simulink model "inverter"  (R2021a)
settings: Solver=VariableStepAuto  StartTime=0.0  StopTime=1  RelTol=1e-3
libraries: spsSeriesRLCBranchLib x2, spsDCVoltageSourceLib x1, spsGroundLib x1, spsThreePhaseParallelRLCBranchLib x1, spsPWMGenerator3LevelLib x1, spsThreeLevelBridgeLib x1, spsThreePhaseVIMeasurementLib x1, spspowerguiLib x1
settings Model: Creator=mluser  LastModifiedBy=mluser

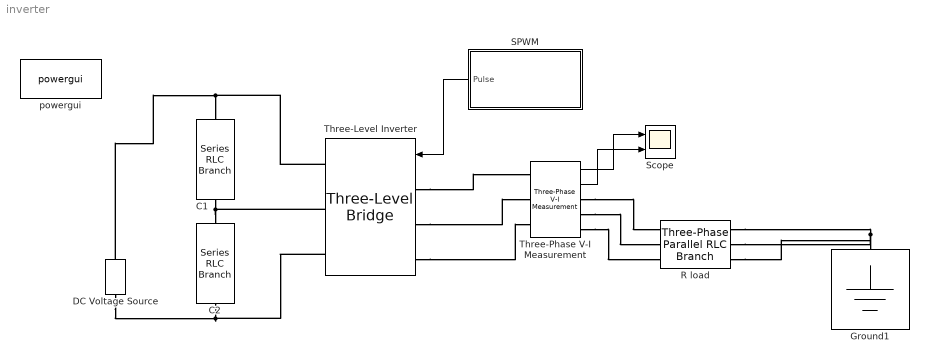
== system inverter ==
  C1 : spsSeriesRLCBranchLib/Series RLC Branch  LConnTagsString=__new0  RConnTagsString=__new0  BranchType=RC  Resistance=1e-3  Inductance=1e-3  SetiL0=off  InitialCurrent=0  Capacitance=3300e-6  Setx0=off  InitialVoltage=0  Measurements=None
  C2 : spsSeriesRLCBranchLib/Series RLC Branch  LConnTagsString=__new0  RConnTagsString=__new0  BranchType=RC  Resistance=1e-3  Inductance=1e-3  SetiL0=off  InitialCurrent=0  Capacitance=3300e-6  Setx0=off  InitialVoltage=0  Measurements=None
  DC Voltage Source : spsDCVoltageSourceLib/DC Voltage Source  Amplitude=230  Measurements=None
  Ground1 : spsGroundLib/Ground  LConnTagsString=a
  R load : spsThreePhaseParallelRLCBranchLib/Three-Phase Parallel RLC Branch  LConnTagsString=A|B|C  RConnTagsString=A|B|C  BranchType=R  Resistance=1e3  Inductance=1e-3  Capacitance=1e-6  Measurements=None
      settings: SourceProductBaseCode=PS
  SPWM : Subsystem
  Scope : Scope  NumInputPorts=2
  Three-Level Inverter : spsThreeLevelBridgeLib/Three-Level Bridge  Arms=3  SnubberResistance=1e5  SbubberCapacitance=inf  Device=IGBT / Diodes  Ron=1e-3  ForwardVoltages="[  0  0  ]"  Measurements=None
      settings: SourceProductBaseCode=PS
  Three-Phase V-I Measurement : spsThreePhaseVIMeasurementLib/Three-Phase V-I Measurement  VoltageMeasurement=phase-to-phase  SetLabelV=off  LabelV=Vabc  Vpu=off  VpuLL=off  CurrentMeasurement=yes  SetLabelI=off  LabelI=Iabc  Ipu=off  Pbase=100e6  Vbase=500e3  OutputType=Complex  PhasorSimulation=off  PSBequivalent=0
  powergui : spspowerguiLib/powergui  Priority=1  SimulationMode=Discrete  SampleTime=1e-6  frequency=60  Iterations=50  frequencyindice=0  Pbase=100e6  ErrMax=1e-4  UnitsV=kV  UnitsW=MW  buscounter=0  FunctionMessages=off  echomessages=off  EnableUseOfTLC=off  CurrentSourceSwitches=off  DisableSnubberDevices=off  DisableRonSwitches=off  DisableVfSwitches=off  DisplayEquations=off  AutomaticDiscreteSolvers=off  SolverType=Tustin/Backward Euler (TBE)  Interpol=off  ExternalGateDelay=off  methode=off  Ts=100  x0status=blocks  SPID=on  SwTol=0  HookPort=off  NonlinearTolerance=1e-4  nMaxIteration=100  ContinueOnMaxIteration=off  RestoreLinks=warning  ResistiveCurrentMeasurement=off  Frange=[0:2:500]  Ylog=off  Xlog=on  ShowGrid=off  save=off  variable=ZData  structure=0  ZoomFFT=off  StartTime=0.0  cycles=1  DisplayStyle=1  fundamental=60  FreqAxis=off  MaxFrequency=1000  frequencyindicesteady=1  RmsSteady=1  display=off
  wires:
  SPWM/1(Pulse) -> Three-Level Inverter/1
  Three-Phase V-I Measurement/1 -> Scope/1
  Three-Phase V-I Measurement/2 -> Scope/2
  connections:
  C2/RConn1 -- DC Voltage Source/LConn1 -- Three-Level Inverter/RConn3
  DC Voltage Source/RConn1 -- Three-Level Inverter/RConn1 -- C1/LConn1
  Three-Level Inverter/RConn2 -- C1/RConn1 -- C2/LConn1
  Three-Level Inverter/LConn1 -- Three-Phase V-I Measurement/LConn1
  Three-Level Inverter/LConn2 -- Three-Phase V-I Measurement/LConn2
  Three-Level Inverter/LConn3 -- Three-Phase V-I Measurement/LConn3
  Three-Phase V-I Measurement/RConn1 -- R load/LConn1
  Three-Phase V-I Measurement/RConn2 -- R load/LConn2
  Three-Phase V-I Measurement/RConn3 -- R load/LConn3
  R load/RConn1 -- R load/RConn3 -- R load/RConn2 -- Ground1/LConn1

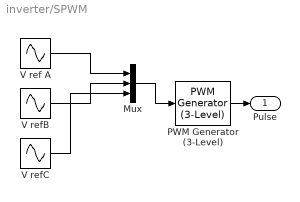
== system inverter/SPWM ==
  Mux : Mux  Inputs=3
  PWM Generator (3-Level) : spsPWMGenerator3LevelLib/PWM Generator (3-Level)  ModulatorType=Three-phase bridge (12 pulses)  ModulatorMode=Unsynchronized  nF=27  Fc=27*50*3  ModulatingSignals=off  m=0.8  Freq=60  Phase=0  Ts=0
      settings: SourceProductBaseCode=PS
  V ref A : Sin  Frequency=2*pi*50  SampleTime=0
  V refB : Sin  Frequency=2*pi*50  Phase=2*pi/3  SampleTime=0
  V refC : Sin  Frequency=2*pi*50  Phase=4*pi/3  SampleTime=0
  Pulse : Outport
  wires:
  V ref A/1 -> Mux/1
  Mux/1 -> PWM Generator (3-Level)/1
  V refC/1 -> Mux/3
  PWM Generator (3-Level)/1 -> Pulse/1
  V refB/1 -> Mux/2
